simulink model "KVHSerial01"  (Simulink 7.9)
settings: Solver=ode45  StartTime=0.0  StopTime=3  RelTol=1e-3
undefined symbols (not defined in the file or in its folder): marlo_lib_v01, serial, SerialIMU
libraries: simulink x2, instrumentlib x2
settings Model: Creator=bgbuss  LastModifiedBy=bgbuss
settings DataIOCC: LimitDataPoints=off

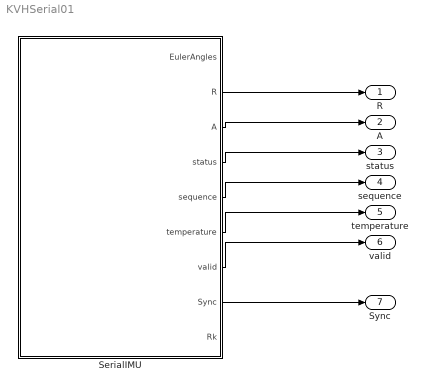
== system KVHSerial01 ==
  SerialIMU : Subsystem  AncestorBlock=marlo_lib_v01/SerialIMU
  R : Outport
  A : Outport  Port=2
  status : Outport  Port=3
  sequence : Outport  Port=4
  temperature : Outport  Port=5
  valid : Outport  Port=6
  Sync : Outport  Port=7
  wires:
  SerialIMU/7(valid) -> valid/1
  SerialIMU/3(A) -> A/1
  SerialIMU/2(R) -> R/1
  SerialIMU/4(status) -> status/1
  SerialIMU/5(sequence) -> sequence/1
  SerialIMU/6(temperature) -> temperature/1
  SerialIMU/8(Sync) -> Sync/1

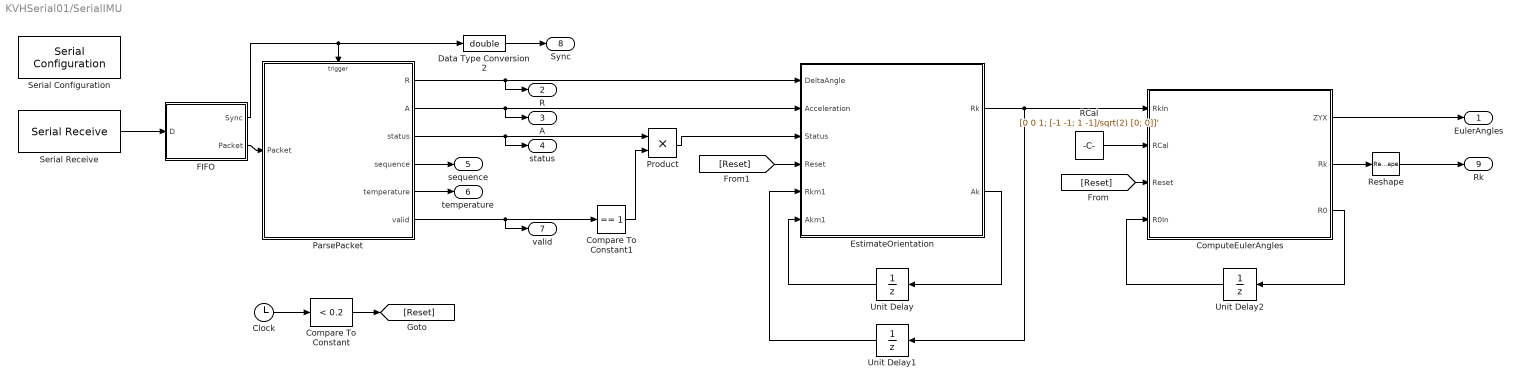
== system KVHSerial01/SerialIMU ==
  Clock : Clock
  Compare To Constant : simulink/Logic and Bit Operations/Compare To Constant  relop=<  const=0.2  OutDataTypeStr=uint8
  Compare To Constant1 : simulink/Logic and Bit Operations/Compare To Constant  relop===  const=1  OutDataTypeStr=uint8
  ComputeEulerAngles : MATLAB Function  TreatAsAtomicUnit=on
  Data Type Conversion2 : DataTypeConversion  OutDataTypeStr=double
  EstimateOrientation : MATLAB Function  TreatAsAtomicUnit=on
  FIFO : Subsystem
  ParsePacket : Subsystem
  Product : Product  RndMeth=Zero
  RCal : Constant  Value=[0 0 1; [-1 -1; 1 -1]/sqrt(2) [0; 0]]'
  Reshape : Reshape
  Serial Configuration : instrumentlib/Serial Configuration  Priority=-200000  ComPortMenu=<Please select a port...>  ComPort=COM5  ObjConstructor=serial('COM5');  BaudRate=460800  DataBits=8  Parity=none  StopBits=1  FlowControl=none  Timeout=10  ByteOrder=LittleEndian
  Serial Receive : instrumentlib/Serial Receive  ComPortMenu=<Please select a port...>  ComPort=COM5  ObjConstructor=serial('COM5');  Terminator=<none>  DataSize=500  DataType=uint8  EnableBlockingMode=on  ActionDataUnavailable=Output last received value  CustomValue=0  SampleTime=0.01
  Unit Delay : UnitDelay  X0=[0; 0; 0]  SampleTime=-1
  Unit Delay1 : UnitDelay  X0=zeros(3,3)  SampleTime=-1
  Unit Delay2 : UnitDelay  X0=zeros(3,3)  SampleTime=-1
  EulerAngles : Outport
  R : Outport  Port=2
  A : Outport  Port=3
  status : Outport  Port=4
  sequence : Outport  Port=5
  temperature : Outport  Port=6
  valid : Outport  Port=7
  Sync : Outport  Port=8
  Rk : Outport  Port=9
  wires:
  ParsePacket/2(A) -> EstimateOrientation/2(Acceleration), A/1
  ParsePacket/1(R) -> EstimateOrientation/1(DeltaAngle), R/1
  Serial Receive/1 -> FIFO/1(D)
  ParsePacket/3(status) -> status/1, Product/1
  ParsePacket/4(sequence) -> sequence/1
  ParsePacket/5(temperature) -> temperature/1
  FIFO/2(Packet) -> ParsePacket/1(Packet)
  FIFO/1(Sync) -> ParsePacket/Trigger, Data Type Conversion2/1
  ParsePacket/6(valid) -> valid/1, Compare To Constant1/1
  Data Type Conversion2/1 -> Sync/1
  EstimateOrientation/2(Ak) -> Unit Delay/1
  Unit Delay/1 -> EstimateOrientation/6(Akm1)
  EstimateOrientation/1(Rk) -> Unit Delay1/1, ComputeEulerAngles/1(RkIn)
  Unit Delay1/1 -> EstimateOrientation/5(Rkm1)
  [Reset] -> EstimateOrientation/4(Reset)
  RCal/1 -> ComputeEulerAngles/2(RCal)
  Unit Delay2/1 -> ComputeEulerAngles/4(R0In)
  ComputeEulerAngles/1(ZYX) -> EulerAngles/1
  ComputeEulerAngles/3(R0) -> Unit Delay2/1
  ComputeEulerAngles/2(Rk) -> Reshape/1
  [Reset] -> ComputeEulerAngles/3(Reset)
  Clock/1 -> Compare To Constant/1
  Compare To Constant/1 -> [Reset]
  Reshape/1 -> Rk/1
  Product/1 -> EstimateOrientation/3(Status)
  Compare To Constant1/1 -> Product/2

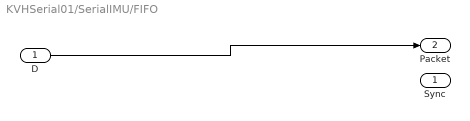
== system KVHSerial01/SerialIMU/FIFO ==
  D : Inport
  Sync : Outport
  Packet : Outport  Port=2
  wires:
  ? -> Sync/1
  D/1 -> Packet/1

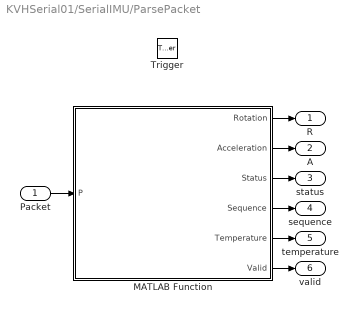
== system KVHSerial01/SerialIMU/ParsePacket ==
  Packet : Inport
  Trigger : TriggerPort  PortDimensions=1
  MATLAB Function : MATLAB Function  TreatAsAtomicUnit=on
  R : Outport
  A : Outport  Port=2
  status : Outport  Port=3
  sequence : Outport  Port=4
  temperature : Outport  Port=5
  valid : Outport  Port=6
  wires:
  MATLAB Function/1(Rotation) -> R/1
  MATLAB Function/2(Acceleration) -> A/1
  MATLAB Function/3(Status) -> status/1
  Packet/1 -> MATLAB Function/1(P)
  MATLAB Function/4(Sequence) -> sequence/1
  MATLAB Function/5(Temperature) -> temperature/1
  MATLAB Function/6(Valid) -> valid/1

== matlab function SerialIMU/ComputeEulerAngles ==
  data: RkIn input double; RCal input double; Reset input double; R0In input double; ZYX output double; Rk output double; R0 output double
function [ZYX, Rk, R0] = fcn(RkIn, RCal, Reset, R0In) %#codegen
    % Convert from IMU frame to robot frame and compute Euler angles. The
    % yaw angle is zeroed whenever (Reset) is true.
        
    if (Reset)
        % Compute the rotation matrix which zeros the initial yaw
        qT0 = M_to_ZYX(RkIn*RCal);
        R0  = Rz(-qT0(1));
    else
        R0 = R0In;
    end
    
    % Transform from IMU to robot frame and zero initial yaw
    Rk = R0*RkIn*RCal;
    
    % Convert Rk to ZYX Euler angles
    ZYX = M_to_ZYX(Rk);
end

function R = Rz(t)
    R = [cos(t) -sin(t) 0; sin(t) cos(t) 0; 0 0 1];
end

== matlab function SerialIMU/EstimateOrientation ==
  data: DeltaAngle input double; Acceleration input double; Status input double; Reset input double; Rk output double; Rkm1 input double; Akm1 input double; Ak output double
function [Rk, Ak] = fcn(DeltaAngle,Acceleration,Status,Reset,Rkm1,Akm1) %#codegen
    [Rk, Ak] = estimateOrientation(DeltaAngle,Acceleration,Rkm1,Akm1,Status,Reset);
end

== matlab function SerialIMU/ParsePacket/MATLAB Function ==
  data: P input double; Rotation output double; Acceleration output double; Status output double; Sequence output double; Temperature output double; Valid output double
function [Rotation,Acceleration,Status,Sequence,Temperature,Valid] = KVHParsePacket(P)
    %#codegen
    CMD = [254; 129; 255; 85]; %hex2dec(['FE';'81';'FF';'55']);
    
    Valid = 0;
    if all(P(1:4) == CMD)
        Valid = kvhCheckCRC(P);
    end
    
    Rotation = parseSingle(P(5:16,:));
    Acceleration = parseSingle(P(17:28,:));
    Status = double(P(29));
    Sequence = double(P(30));
    Temperature = parseInt16(P(31:32));
end

function S = parseSingle(D)
    Stmp1 = uint32(reshape(D,4,[]));
    Stmp2 = 16777216*Stmp1(1,:) + 65536*Stmp1(2,:) + 256*Stmp1(3,:) + Stmp1(4,:);
    Stmp3 = typecast(Stmp2,'single');
    S = double(Stmp3');
end

function S = parseInt16(D)
    Stmp1 = uint16(reshape(D,2,[]));
    Stmp2 = 256*Stmp1(1,:) + Stmp1(2,:);
    S = double(Stmp2');
end
